simulink library "DT_Library"  (R2025b)
settings: Solver=VariableStepAuto  StartTime=0.0  StopTime=10.0  RelTol=1e-3
undefined symbols (not defined in the file or in its folder): Ala, Arg, Asn, Asp, BMedia, BRX, Choline, CMP, Glc, Glu, Gly, GMP, GSmode, His, Ile, K_ht, K_lt, Lac, Leu, Lys, mAb, Met, Phe, Pro, Ser, Thr, Trp, Tyr, V1, Val, Xv
libraries: simulink x23, $bdroot x15
(part 1 of 2)
settings Model: Creator=fenix  LastModifiedBy=Fenix

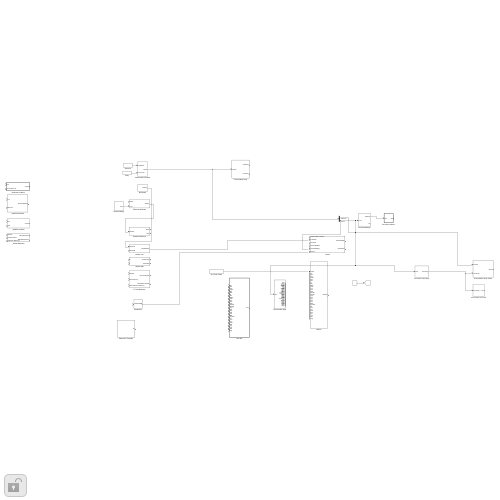
[thumbnail: Simulink's stored preview of the top-level diagram]
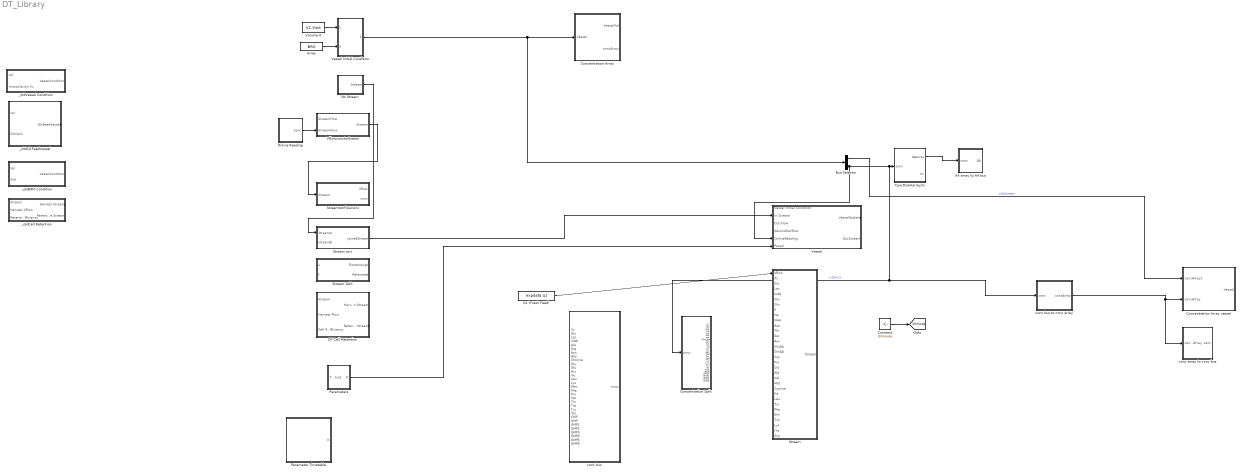
== system DT_Library ==
  AA array to AA bus : Subsystem  TreatAsAtomicUnit=on
  Array : FromWorkspace  VariableName=BRX
  Bus Selector : BusSelector  OutputSignals=Volume,conc
  Concentration Array : Subsystem
  Concentration Array vessel : Subsystem
  Concentration Split : Subsystem
  ConcttoAAarrayXv : Subsystem
  Constant : Constant  Value=GSmode
  DT Cell Retention : Subsystem
  No Stream : Subsystem
  Online Reading : Subsystem
  Parameter Timetable : Subsystem
  Parameters : Subsystem
  Q1 (Fresh Feed) : FromWorkspace  VariableName=expdata.q1  Interpolate=off  OutputAfterFinalValue=Holding final value
  Stream : Subsystem
  Stream Join : Subsystem
  Stream Split : Subsystem
  StreamtoVflowconc : Subsystem
  Vessel : Subsystem
  Vessel Initial Condition : Subsystem
  VflowconctoStream : Subsystem
  Volume 0 : Constant  Value=V1.Vinit
  _oldBRX Condition : Subsystem
  _oldCell Retention : Subsystem
  _oldGlcFeedVessel : Subsystem
  _oldVessel Condition : Subsystem  TreatAsAtomicUnit=on
  conc array to conc bus : Subsystem
  conc bus : Subsystem  TreatAsAtomicUnit=on
  conc bus to conc array : Subsystem
  tag scope: GSmode=global
  wires:
  VflowconctoStream/1(Stream) -> StreamtoVflowconc/1(Stream)
  Stream Join/1(joinedStream) -> Vessel/2(In Stream)
  No Stream/1(Stream) -> Stream Join/1(streamA)
  Array/1 -> Vessel Initial Condition/2(conc array)
  Vessel Initial Condition/1(vessel) -> Bus Selector/1, Concentration Array/1(Vessel)
  Volume 0/1 -> Vessel Initial Condition/1(VesselVol)
  Bus Selector/2 -> Vessel/5(OnlineReading), conc bus to conc array/1(conc), Concentration Split/1(conc), ConcttoAAarrayXv/1(conc)  "<conc>"
  conc bus to conc array/1(concArray) -> conc array to conc bus/1(concArray), Concentration Array vessel/2(concArray)
  Bus Selector/1 -> Concentration Array vessel/1(concArray1)  "<Volume>"
  ConcttoAAarrayXv/1(AAarray) -> AA array to AA bus/1(conc)
  Q1 (Fresh Feed)/1 -> Stream/1(Vflow)
  Parameters/1(K) -> Vessel/6(Param)
  Online Reading/1(conc) -> VflowconctoStream/2(StreamConc)
  Constant/1 -> [GSmode]

== system DT_Library/AA array to AA bus ==
  conc : Inport
  Bus Creator : BusCreator  Inputs=22  OutDataTypeStr=Bus: AA
      settings: InheritFromInputs=off
  Demux : Demux  Outputs=22
  AA : Outport
  wires:
  Demux/1 -> Bus Creator/1
  Demux/2 -> Bus Creator/2
  Demux/3 -> Bus Creator/3
  Demux/4 -> Bus Creator/4
  Demux/5 -> Bus Creator/5
  Demux/6 -> Bus Creator/6
  Demux/7 -> Bus Creator/7
  Demux/8 -> Bus Creator/8
  Demux/9 -> Bus Creator/9
  Demux/10 -> Bus Creator/10
  Demux/11 -> Bus Creator/11
  Demux/12 -> Bus Creator/12
  Demux/13 -> Bus Creator/13
  Demux/14 -> Bus Creator/14
  Demux/15 -> Bus Creator/15
  Demux/16 -> Bus Creator/16
  Demux/17 -> Bus Creator/17
  Demux/18 -> Bus Creator/18
  Demux/19 -> Bus Creator/19
  Demux/20 -> Bus Creator/20
  Demux/21 -> Bus Creator/21
  Bus Creator/1 -> AA/1
  conc/1 -> Demux/1
  Demux/22 -> Bus Creator/22

== system DT_Library/Concentration Array ==
  Vessel : Inport  OutDataTypeStr=Bus: Vessel
  Bus Selector : BusSelector  OutputSignals=Volume,conc
  conc bus to conc array : $bdroot/conc bus to conc array  SystemSampleTime=-1  VariantActivationTime=update diagram  EmptyChoice=off  PassThrough=off  PassThroughVariantControl=(default)  EmptyChoiceVariantControl=(default)  AllowFlexibleInterface=on  Latency=0  AutoFrameSizeCalculation=off
  VesselVol : Outport  OutDataTypeStr=ValueType: Volume
  concArray : Outport  Port=2
  wires:
  Bus Selector/2 -> conc bus to conc array/1  "<conc>"
  Vessel/1 -> Bus Selector/1
  Bus Selector/1 -> VesselVol/1  "<Volume>"
  conc bus to conc array/1 -> concArray/1

== system DT_Library/Concentration Array vessel ==
  concArray1 : Inport
  concArray : Inport  Port=2
  Bus Creator : BusCreator  Inputs=2  OutDataTypeStr=Bus: Vessel  NonVirtualBus=on
  conc array to conc bus : $bdroot/conc array to conc bus  SystemSampleTime=-1  VariantActivationTime=update diagram  EmptyChoice=off  PassThrough=off  PassThroughVariantControl=(default)  EmptyChoiceVariantControl=(default)  AllowFlexibleInterface=on  Latency=0  AutoFrameSizeCalculation=off
  Vessel : Outport  OutDataTypeStr=Bus: Vessel
  wires:
  concArray1/1 -> Bus Creator/1  "Volume"
  Bus Creator/1 -> Vessel/1
  concArray/1 -> conc array to conc bus/1  "concArray"
  conc array to conc bus/1 -> Bus Creator/2  "conc"

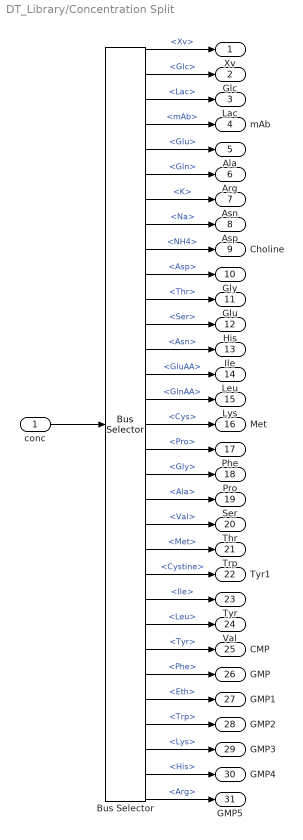
== system DT_Library/Concentration Split ==
  conc : Inport  OutDataTypeStr=Bus: conc
  Bus Selector : BusSelector  OutputSignals=Xv,Glc,Lac,mAb,Glu,Gln,K,Na,NH4,Asp,Thr,Ser,Asn,GluAA,GlnAA,Cys,Pro,Gly,Ala,Val,Met,Cystine,Ile,Leu,Tyr,Phe,Eth,Trp,Lys,His,Arg
  Xv : Outport  OutDataTypeStr=ValueType: Xvconc
  Glc : Outport  Port=2  OutDataTypeStr=ValueType: gconc
  Lac : Outport  Port=3  OutDataTypeStr=ValueType: gconc
  mAb : Outport  Port=4  OutDataTypeStr=ValueType: gconc
  Ala : Outport  Port=5  OutDataTypeStr=ValueType: mMconc
  Arg : Outport  Port=6  OutDataTypeStr=ValueType: mMconc
  Asn : Outport  Port=7  OutDataTypeStr=ValueType: mMconc
  Asp : Outport  Port=8  OutDataTypeStr=ValueType: mMconc
  Choline : Outport  Port=9  OutDataTypeStr=ValueType: mMconc
  Gly : Outport  Port=10  OutDataTypeStr=ValueType: mMconc
  Glu : Outport  Port=11  OutDataTypeStr=ValueType: mMconc
  His : Outport  Port=12  OutDataTypeStr=ValueType: mMconc
  Ile : Outport  Port=13  OutDataTypeStr=ValueType: mMconc
  Leu : Outport  Port=14  OutDataTypeStr=ValueType: mMconc
  Lys : Outport  Port=15  OutDataTypeStr=ValueType: mMconc
  Met : Outport  Port=16  OutDataTypeStr=ValueType: mMconc
  Phe : Outport  Port=17  OutDataTypeStr=ValueType: mMconc
  Pro : Outport  Port=18  OutDataTypeStr=ValueType: mMconc
  Ser : Outport  Port=19  OutDataTypeStr=ValueType: mMconc
  Thr : Outport  Port=20  OutDataTypeStr=ValueType: mMconc
  Trp : Outport  Port=21  OutDataTypeStr=ValueType: mMconc
  Tyr1 : Outport  Port=22  OutDataTypeStr=ValueType: mMconc
  Tyr : Outport  Port=23  OutDataTypeStr=ValueType: mMconc
  Val : Outport  Port=24  OutDataTypeStr=ValueType: mMconc
  CMP : Outport  Port=25  OutDataTypeStr=ValueType: mMconc
  GMP : Outport  Port=26  OutDataTypeStr=ValueType: mMconc
  GMP1 : Outport  Port=27  OutDataTypeStr=ValueType: mMconc
  GMP2 : Outport  Port=28  OutDataTypeStr=ValueType: mMconc
  GMP3 : Outport  Port=29  OutDataTypeStr=ValueType: mMconc
  GMP4 : Outport  Port=30  OutDataTypeStr=ValueType: mMconc
  GMP5 : Outport  Port=31  OutDataTypeStr=ValueType: mMconc
  wires:
  conc/1 -> Bus Selector/1
  Bus Selector/2 -> Glc/1  "<Glc>"
  Bus Selector/4 -> mAb/1  "<mAb>"
  Bus Selector/3 -> Lac/1  "<Lac>"
  Bus Selector/8 -> Asp/1  "<Na>"
  Bus Selector/16 -> Met/1  "<Cys>"
  Bus Selector/15 -> Lys/1  "<GlnAA>"
  Bus Selector/14 -> Leu/1  "<GluAA>"
  Bus Selector/13 -> Ile/1  "<Asn>"
  Bus Selector/12 -> His/1  "<Ser>"
  Bus Selector/11 -> Glu/1  "<Thr>"
  Bus Selector/10 -> Gly/1  "<Asp>"
  Bus Selector/9 -> Choline/1  "<NH4>"
  Bus Selector/5 -> Ala/1  "<Glu>"
  Bus Selector/6 -> Arg/1  "<Gln>"
  Bus Selector/7 -> Asn/1  "<K>"
  Bus Selector/21 -> Trp/1  "<Met>"
  Bus Selector/20 -> Thr/1  "<Val>"
  Bus Selector/19 -> Ser/1  "<Ala>"
  Bus Selector/18 -> Pro/1  "<Gly>"
  Bus Selector/17 -> Phe/1  "<Pro>"
  Bus Selector/1 -> Xv/1  "<Xv>"
  Bus Selector/24 -> Val/1  "<Leu>"
  Bus Selector/25 -> CMP/1  "<Tyr>"
  Bus Selector/26 -> GMP/1  "<Phe>"
  Bus Selector/23 -> Tyr/1  "<Ile>"
  Bus Selector/22 -> Tyr1/1  "<Cystine>"
  Bus Selector/27 -> GMP1/1  "<Eth>"
  Bus Selector/31 -> GMP5/1  "<Arg>"
  Bus Selector/30 -> GMP4/1  "<His>"
  Bus Selector/29 -> GMP3/1  "<Lys>"
  Bus Selector/28 -> GMP2/1  "<Trp>"

== system DT_Library/ConcttoAAarrayXv ==
  conc : Inport
  Concentration Split : $bdroot/Concentration Split  SystemSampleTime=-1  VariantActivationTime=update diagram  EmptyChoice=off  PassThrough=off  PassThroughVariantControl=(default)  EmptyChoiceVariantControl=(default)  AllowFlexibleInterface=on  Latency=0  AutoFrameSizeCalculation=off
  Mux : Mux  Inputs=22
  AAarray : Outport
  Xv : Outport  Port=2
  wires:
  conc/1 -> Concentration Split/1
  Mux/1 -> AAarray/1
  Concentration Split/1 -> Xv/1
  Concentration Split/10 -> Mux/1
  Concentration Split/11 -> Mux/2
  Concentration Split/12 -> Mux/3
  Concentration Split/13 -> Mux/4
  Concentration Split/14 -> Mux/5
  Concentration Split/15 -> Mux/6
  Concentration Split/16 -> Mux/7
  Concentration Split/17 -> Mux/8
  Concentration Split/18 -> Mux/9
  Concentration Split/19 -> Mux/10
  Concentration Split/20 -> Mux/11
  Concentration Split/21 -> Mux/12
  Concentration Split/22 -> Mux/13
  Concentration Split/23 -> Mux/14
  Concentration Split/24 -> Mux/15
  Concentration Split/25 -> Mux/16
  Concentration Split/26 -> Mux/17
  Concentration Split/27 -> Mux/18
  Concentration Split/28 -> Mux/19
  Concentration Split/29 -> Mux/20
  Concentration Split/30 -> Mux/21
  Concentration Split/31 -> Mux/22

== system DT_Library/DT Cell Retention ==
  Stream : Inport  OutDataTypeStr=Bus: Stream
  Harvest Flow : Inport  Port=2  OutDataTypeStr=ValueType: Flow
  Cell Retention Efficiency : Inport  Port=3
  CellRet : MATLAB Function  TreatAsAtomicUnit=on
  Harvest Stream : Outport  OutDataTypeStr=Bus: Stream
  Retentation Stream : Outport  Port=2  OutDataTypeStr=Bus: Stream
  wires:
  Cell Retention Efficiency/1 -> CellRet/3(RetEff)
  Harvest Flow/1 -> CellRet/2(HarvFlow)
  Stream/1 -> CellRet/1(Stream)
  CellRet/2(Ret_Stream) -> Retentation Stream/1
  CellRet/1(Harv_Stream) -> Harvest Stream/1

== system DT_Library/No Stream ==
  Stream1 : $bdroot/Stream  SystemSampleTime=-1  VariantActivationTime=update diagram  EmptyChoice=off  PassThrough=off  PassThroughVariantControl=(default)  EmptyChoiceVariantControl=(default)  AllowFlexibleInterface=on  Latency=0  AutoFrameSizeCalculation=off
  zeroXv : Constant  Value=0  OutDataTypeStr=ValueType: Xvconc
  zeroflow : Constant  Value=0  OutDataTypeStr=ValueType: Flow
  zerogconc : Constant  Value=0  OutDataTypeStr=ValueType: gconc
  zeromM : Constant  Value=0  OutDataTypeStr=ValueType: mMconc
  Stream : Outport  OutDataTypeStr=Bus: Stream
  wires:
  Stream1/1 -> Stream/1
  zeroflow/1 -> Stream1/1
  zeroXv/1 -> Stream1/2
  zerogconc/1 -> Stream1/3, Stream1/5, Stream1/4
  zeromM/1 -> Stream1/32, Stream1/31, Stream1/30, Stream1/29, Stream1/28, Stream1/27, Stream1/26, Stream1/25, Stream1/24, Stream1/23, Stream1/22, Stream1/21, Stream1/20, Stream1/19, Stream1/18, Stream1/17, Stream1/16, Stream1/15, Stream1/14, Stream1/13, Stream1/12, Stream1/11, Stream1/10, Stream1/9, Stream1/8, Stream1/7, Stream1/6

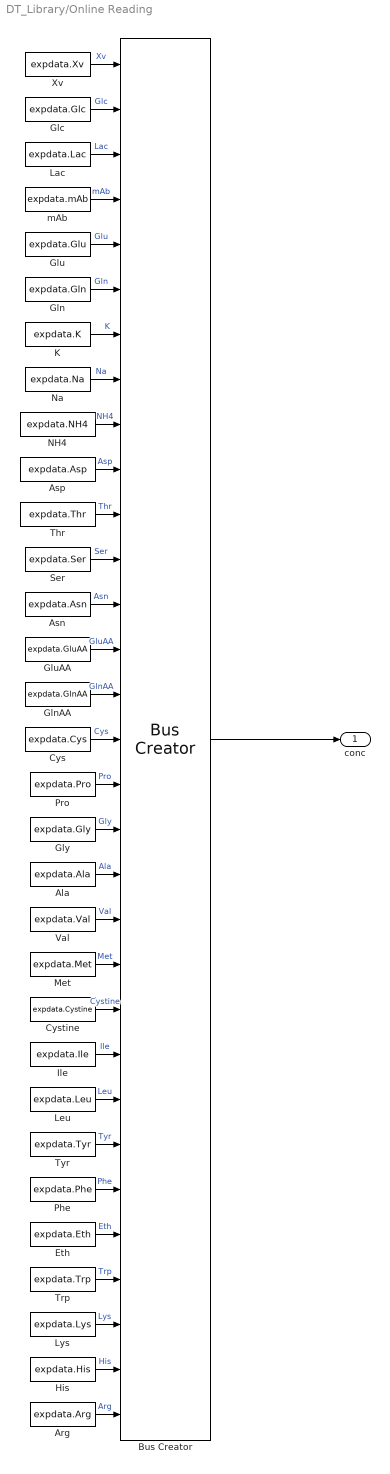
== system DT_Library/Online Reading ==
  "Ala " : FromWorkspace  VariableName=expdata.Ala
  "Arg " : FromWorkspace  VariableName=expdata.Arg
  "Asn " : FromWorkspace  VariableName=expdata.Asn
  "Asp " : FromWorkspace  VariableName=expdata.Asp
  Bus Creator : BusCreator  Inputs=31  OutDataTypeStr=Bus: conc
      settings: InheritFromInputs=off
  "Cys " : FromWorkspace  VariableName=expdata.Cys
  "Cystine " : FromWorkspace  VariableName=expdata.Cystine
  "Eth " : FromWorkspace  VariableName=expdata.Eth
  Glc : FromWorkspace  VariableName=expdata.Glc
  "Gln " : FromWorkspace  VariableName=expdata.Gln
  "GlnAA " : FromWorkspace  VariableName=expdata.GlnAA
  "Glu " : FromWorkspace  VariableName=expdata.Glu
  "GluAA " : FromWorkspace  VariableName=expdata.GluAA
  "Gly " : FromWorkspace  VariableName=expdata.Gly
  "His " : FromWorkspace  VariableName=expdata.His
  "Ile " : FromWorkspace  VariableName=expdata.Ile
  "K " : FromWorkspace  VariableName=expdata.K
  Lac : FromWorkspace  VariableName=expdata.Lac
  "Leu " : FromWorkspace  VariableName=expdata.Leu
  "Lys " : FromWorkspace  VariableName=expdata.Lys
  "Met " : FromWorkspace  VariableName=expdata.Met
  "NH4 " : FromWorkspace  VariableName=expdata.NH4
  "Na " : FromWorkspace  VariableName=expdata.Na
  Phe : FromWorkspace  VariableName=expdata.Phe
  "Pro " : FromWorkspace  VariableName=expdata.Pro
  "Ser " : FromWorkspace  VariableName=expdata.Ser
  "Thr " : FromWorkspace  VariableName=expdata.Thr
  "Trp " : FromWorkspace  VariableName=expdata.Trp
  Tyr : FromWorkspace  VariableName=expdata.Tyr
  "Val " : FromWorkspace  VariableName=expdata.Val
  Xv : FromWorkspace  VariableName=expdata.Xv
  mAb : FromWorkspace  VariableName=expdata.mAb
  conc : Outport  OutDataTypeStr=Bus: conc
  wires:
  "Glu "/1 -> Bus Creator/5  "Glu"
  "Gln "/1 -> Bus Creator/6  "Gln"
  "K "/1 -> Bus Creator/7  "K"
  "Na "/1 -> Bus Creator/8  "Na"
  Xv/1 -> Bus Creator/1  "Xv"
  Glc/1 -> Bus Creator/2  "Glc"
  Lac/1 -> Bus Creator/3  "Lac"
  mAb/1 -> Bus Creator/4  "mAb"
  Bus Creator/1 -> conc/1
  "NH4 "/1 -> Bus Creator/9  "NH4"
  "Asp "/1 -> Bus Creator/10  "Asp"
  "Thr "/1 -> Bus Creator/11  "Thr"
  "Asn "/1 -> Bus Creator/13  "Asn"
  "Ser "/1 -> Bus Creator/12  "Ser"
  "Eth "/1 -> Bus Creator/27  "Eth"
  Phe/1 -> Bus Creator/26  "Phe"
  Tyr/1 -> Bus Creator/25  "Tyr"
  "Leu "/1 -> Bus Creator/24  "Leu"
  "Ile "/1 -> Bus Creator/23  "Ile"
  "Cystine "/1 -> Bus Creator/22  "Cystine"
  "Met "/1 -> Bus Creator/21  "Met"
  "Val "/1 -> Bus Creator/20  "Val"
  "Ala "/1 -> Bus Creator/19  "Ala"
  "Gly "/1 -> Bus Creator/18  "Gly"
  "Pro "/1 -> Bus Creator/17  "Pro"
  "Cys "/1 -> Bus Creator/16  "Cys"
  "GlnAA "/1 -> Bus Creator/15  "GlnAA"
  "GluAA "/1 -> Bus Creator/14  "GluAA"
  "Arg "/1 -> Bus Creator/31  "Arg"
  "His "/1 -> Bus Creator/30  "His"
  "Lys "/1 -> Bus Creator/29  "Lys"
  "Trp "/1 -> Bus Creator/28  "Trp"

== system DT_Library/Parameter Timetable ==
  From Workspace : FromWorkspace  VariableName=KTT.Ylacglc  Interpolate=off  OutputAfterFinalValue=Holding final value
  From Workspace1 : FromWorkspace  VariableName=KTT.Ymabxv  OutputAfterFinalValue=Holding final value
  From Workspace2 : FromWorkspace  VariableName=KTT.Yxvglc  OutputAfterFinalValue=Holding final value
  From Workspace3 : FromWorkspace  VariableName=KTT.kdlac  OutputAfterFinalValue=Holding final value
  From Workspace4 : FromWorkspace  VariableName=KTT.kglc  OutputAfterFinalValue=Holding final value
  From Workspace5 : FromWorkspace  VariableName=KTT.kilac  OutputAfterFinalValue=Holding final value
  From Workspace6 : FromWorkspace  VariableName=KTT.mglc  OutputAfterFinalValue=Holding final value
  From Workspace7 : FromWorkspace  VariableName=KTT.udmax
  From Workspace8 : FromWorkspace  VariableName=KTT.umax  OutputAfterFinalValue=Holding final value
  From Workspace9 : FromWorkspace  VariableName=KTT.Yxvlac  OutputAfterFinalValue=Holding final value
  parameter bus : $bdroot/Parameters/parameter bus  SystemSampleTime=-1  VariantActivationTime=update diagram  EmptyChoice=off  PassThrough=off  PassThroughVariantControl=(default)  EmptyChoiceVariantControl=(default)  AllowFlexibleInterface=on  Latency=0  AutoFrameSizeCalculation=off
  K : Outport
  wires:
  From Workspace2/1 -> parameter bus/3
  From Workspace9/1 -> parameter bus/10
  From Workspace/1 -> parameter bus/1
  From Workspace3/1 -> parameter bus/4
  From Workspace1/1 -> parameter bus/2
  From Workspace6/1 -> parameter bus/7
  From Workspace4/1 -> parameter bus/5
  From Workspace8/1 -> parameter bus/9
  From Workspace5/1 -> parameter bus/6
  From Workspace7/1 -> parameter bus/8
  parameter bus/1 -> K/1

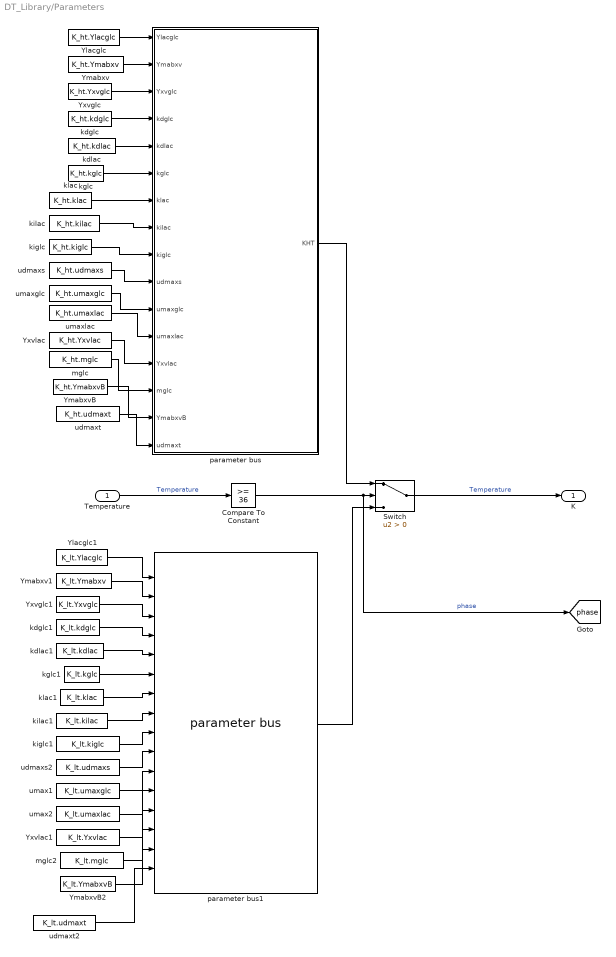
== system DT_Library/Parameters ==
  Temperature : Inport
  Compare To Constant : simulink/Logic and Bit Operations/Compare To Constant  relop=>=  const=36  OutDataTypeStr=boolean
  Switch : Switch  Criteria=u2 > Threshold  ZeroCross=off  SaturateOnIntegerOverflow=off  InputSameDT=off
  Ylacglc : Constant  Value=K_ht.Ylacglc
  Ylacglc1 : Constant  Value=K_lt.Ylacglc
  Ymabxv : Constant  Value=K_ht.Ymabxv
  Ymabxv1 : Constant  Value=K_lt.Ymabxv
  YmabxvB : Constant  Value=K_ht.YmabxvB
  YmabxvB2 : Constant  Value=K_lt.YmabxvB
  Yxvglc : Constant  Value=K_ht.Yxvglc
  Yxvglc1 : Constant  Value=K_lt.Yxvglc
  Yxvlac : Constant  Value=K_ht.Yxvlac
  Yxvlac1 : Constant  Value=K_lt.Yxvlac
  kdglc : Constant  Value=K_ht.kdglc
  kdglc1 : Constant  Value=K_lt.kdglc
  kdlac : Constant  Value=K_ht.kdlac
  kdlac1 : Constant  Value=K_lt.kdlac
  kglc : Constant  Value=K_ht.kglc
  kglc1 : Constant  Value=K_lt.kglc
  kiglc : Constant  Value=K_ht.kiglc
  kiglc1 : Constant  Value=K_lt.kiglc
  kilac : Constant  Value=K_ht.kilac
  kilac1 : Constant  Value=K_lt.kilac
  klac : Constant  Value=K_ht.klac
  klac1 : Constant  Value=K_lt.klac
  mglc : Constant  Value=K_ht.mglc
  mglc2 : Constant  Value=K_lt.mglc
  parameter bus : Subsystem  TreatAsAtomicUnit=on
  parameter bus1 : $bdroot/Parameters/parameter bus  SystemSampleTime=-1  VariantActivationTime=update diagram  EmptyChoice=off  PassThrough=off  PassThroughVariantControl=(default)  EmptyChoiceVariantControl=(default)  AllowFlexibleInterface=on  Latency=0  AutoFrameSizeCalculation=off
  udmaxs : Constant  Value=K_ht.udmaxs
  udmaxs2 : Constant  Value=K_lt.udmaxs
  udmaxt : Constant  Value=K_ht.udmaxt
  udmaxt2 : Constant  Value=K_lt.udmaxt
  umax1 : Constant  Value=K_lt.umaxglc
  umax2 : Constant  Value=K_lt.umaxlac
  umaxglc : Constant  Value=K_ht.umaxglc
  umaxlac : Constant  Value=K_ht.umaxlac
  K : Outport
  tag scope: phase=global
  wires:
  parameter bus/1(KHT) -> Switch/1
  kdlac/1 -> parameter bus/5(kdlac)
  Ylacglc/1 -> parameter bus/1(Ylacglc)
  kglc/1 -> parameter bus/6(kglc)
  Ymabxv/1 -> parameter bus/2(Ymabxv)
  klac/1 -> parameter bus/7(klac)
  Yxvglc/1 -> parameter bus/3(Yxvglc)
  kilac/1 -> parameter bus/8(kilac)
  kdglc/1 -> parameter bus/4(kdglc)
  kiglc/1 -> parameter bus/9(kiglc)
  Temperature/1 -> Compare To Constant/1  "Temperature"
  Compare To Constant/1 -> [phase], Switch/2  "phase"
  parameter bus1/1 -> Switch/3
  Switch/1 -> K/1  "Temperature"
  udmaxs/1 -> parameter bus/10(udmaxs)
  umaxglc/1 -> parameter bus/11(umaxglc)
  umaxlac/1 -> parameter bus/12(umaxlac)
  Ylacglc1/1 -> parameter bus1/1
  Ymabxv1/1 -> parameter bus1/2
  Yxvglc1/1 -> parameter bus1/3
  kdglc1/1 -> parameter bus1/4
  kdlac1/1 -> parameter bus1/5
  kglc1/1 -> parameter bus1/6
  kilac1/1 -> parameter bus1/8
  klac1/1 -> parameter bus1/7
  kiglc1/1 -> parameter bus1/9
  udmaxs2/1 -> parameter bus1/10
  umax1/1 -> parameter bus1/11
  Yxvlac/1 -> parameter bus/13(Yxvlac)
  mglc/1 -> parameter bus/14(mglc)
  YmabxvB/1 -> parameter bus/15(YmabxvB)
  Yxvlac1/1 -> parameter bus1/13
  umax2/1 -> parameter bus1/12
  YmabxvB2/1 -> parameter bus1/15
  mglc2/1 -> parameter bus1/14
  udmaxt2/1 -> parameter bus1/16
  udmaxt/1 -> parameter bus/16(udmaxt)

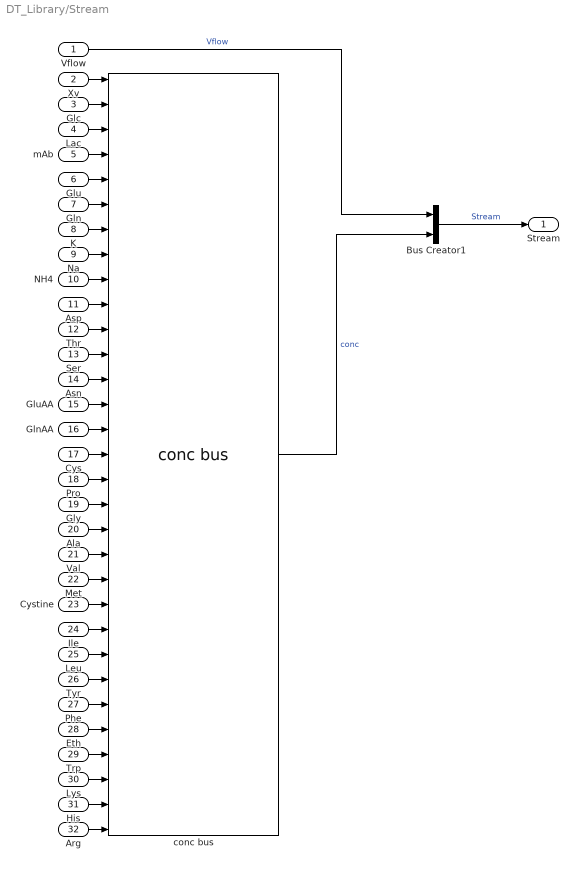
== system DT_Library/Stream ==
  Vflow : Inport  OutDataTypeStr=ValueType: Flow
  "Xv " : Inport  Port=2  OutDataTypeStr=ValueType: Xvconc
  "Glc " : Inport  Port=3  OutDataTypeStr=ValueType: gconc
  "Lac " : Inport  Port=4  OutDataTypeStr=ValueType: gconc
  mAb : Inport  Port=5  OutDataTypeStr=ValueType: gconc
  "Glu " : Inport  Port=6  OutDataTypeStr=ValueType: mMconc
  "Gln " : Inport  Port=7  OutDataTypeStr=ValueType: mMconc
  "K " : Inport  Port=8  OutDataTypeStr=ValueType: mMconc
  "Na " : Inport  Port=9  OutDataTypeStr=ValueType: mMconc
  "NH4 " : Inport  Port=10  OutDataTypeStr=ValueType: mMconc
  "Asp " : Inport  Port=11  OutDataTypeStr=ValueType: mMconc
  "Thr " : Inport  Port=12  OutDataTypeStr=ValueType: mMconc
  "Ser " : Inport  Port=13  OutDataTypeStr=ValueType: mMconc
  "Asn " : Inport  Port=14  OutDataTypeStr=ValueType: mMconc
  "GluAA " : Inport  Port=15  OutDataTypeStr=ValueType: mMconc
  "GlnAA " : Inport  Port=16  OutDataTypeStr=ValueType: mMconc
  "Cys " : Inport  Port=17  OutDataTypeStr=ValueType: mMconc
  "Pro " : Inport  Port=18  OutDataTypeStr=ValueType: mMconc
  "Gly " : Inport  Port=19  OutDataTypeStr=ValueType: mMconc
  "Ala " : Inport  Port=20  OutDataTypeStr=ValueType: mMconc
  "Val " : Inport  Port=21  OutDataTypeStr=ValueType: mMconc
  "Met " : Inport  Port=22  OutDataTypeStr=ValueType: mMconc
  "Cystine " : Inport  Port=23  OutDataTypeStr=ValueType: mMconc
  "Ile " : Inport  Port=24  OutDataTypeStr=ValueType: mMconc
  "Leu " : Inport  Port=25  OutDataTypeStr=ValueType: mMconc
  "Tyr " : Inport  Port=26  OutDataTypeStr=ValueType: mMconc
  "Phe " : Inport  Port=27  OutDataTypeStr=ValueType: mMconc
  "Eth " : Inport  Port=28  OutDataTypeStr=ValueType: mMconc
  "Trp " : Inport  Port=29  OutDataTypeStr=ValueType: mMconc
  "Lys " : Inport  Port=30  OutDataTypeStr=ValueType: mMconc
  "His " : Inport  Port=31  OutDataTypeStr=ValueType: mMconc
  "Arg " : Inport  Port=32  OutDataTypeStr=ValueType: mMconc
  Bus Creator1 : BusCreator  Inputs=2  OutDataTypeStr=Bus: Stream
      settings: InheritFromInputs=off
  conc bus : $bdroot/conc bus  SystemSampleTime=-1  VariantActivationTime=update diagram  EmptyChoice=off  PassThrough=off  PassThroughVariantControl=(default)  EmptyChoiceVariantControl=(default)  AllowFlexibleInterface=on  Latency=0  AutoFrameSizeCalculation=off
  Stream : Outport  OutDataTypeStr=Bus: Stream
  wires:
  Vflow/1 -> Bus Creator1/1  "Vflow"
  Bus Creator1/1 -> Stream/1  "Stream"
  conc bus/1 -> Bus Creator1/2  "conc"
  "Xv "/1 -> conc bus/1
  "Lac "/1 -> conc bus/3
  "Glc "/1 -> conc bus/2
  mAb/1 -> conc bus/4
  "Glu "/1 -> conc bus/5
  "Gln "/1 -> conc bus/6
  "Ala "/1 -> conc bus/19
  "Arg "/1 -> conc bus/31
  "His "/1 -> conc bus/30
  "Lys "/1 -> conc bus/29
  "Trp "/1 -> conc bus/28
  "Eth "/1 -> conc bus/27
  "Phe "/1 -> conc bus/26
  "Tyr "/1 -> conc bus/25
  "Leu "/1 -> conc bus/24
  "Ile "/1 -> conc bus/23
  "Cystine "/1 -> conc bus/22
  "Met "/1 -> conc bus/21
  "Val "/1 -> conc bus/20
  "Gly "/1 -> conc bus/18
  "Pro "/1 -> conc bus/17
  "Cys "/1 -> conc bus/16
  "GlnAA "/1 -> conc bus/15
  "GluAA "/1 -> conc bus/14
  "Asn "/1 -> conc bus/13
  "Ser "/1 -> conc bus/12
  "Thr "/1 -> conc bus/11
  "Asp "/1 -> conc bus/10
  "NH4 "/1 -> conc bus/9
  "Na "/1 -> conc bus/8
  "K "/1 -> conc bus/7

== system DT_Library/Stream Join ==
  streamA : Inport  OutDataTypeStr=Bus: Stream
  streamB : Inport  Port=2  OutDataTypeStr=Bus: Stream
  MATLAB Function : MATLAB Function  TreatAsAtomicUnit=on
  joinedStream : Outport  OutDataTypeStr=Bus: Stream
  wires:
  streamB/1 -> MATLAB Function/2(B)
  streamA/1 -> MATLAB Function/1(A)
  MATLAB Function/1(joinedstream) -> joinedStream/1

== system DT_Library/Stream Split ==
  u : Inport  OutDataTypeStr=Bus: Stream
  f : Inport  Port=2  OutDataTypeStr=Bus: Stream
  MATLAB Function : MATLAB Function  TreatAsAtomicUnit=on
  Flowthrough : Outport  OutDataTypeStr=Bus: Stream
  Retentate : Outport  Port=2  OutDataTypeStr=Bus: Stream
  wires:
  MATLAB Function/1(Flowthrough) -> Flowthrough/1
  MATLAB Function/2(Retentate) -> Retentate/1
  u/1 -> MATLAB Function/1(u)
  f/1 -> MATLAB Function/2(f)

== system DT_Library/StreamtoVflowconc ==
  Stream : Inport  OutDataTypeStr=Bus: Stream
  Bus Selector : BusSelector  OutputSignals=Vflow,conc
  Vflow : Outport  OutDataTypeStr=ValueType: Flow
  conc : Outport  Port=2  OutDataTypeStr=Bus: conc
  wires:
  Stream/1 -> Bus Selector/1
  Bus Selector/1 -> Vflow/1  "<Vflow>"
  Bus Selector/2 -> conc/1  "<conc>"

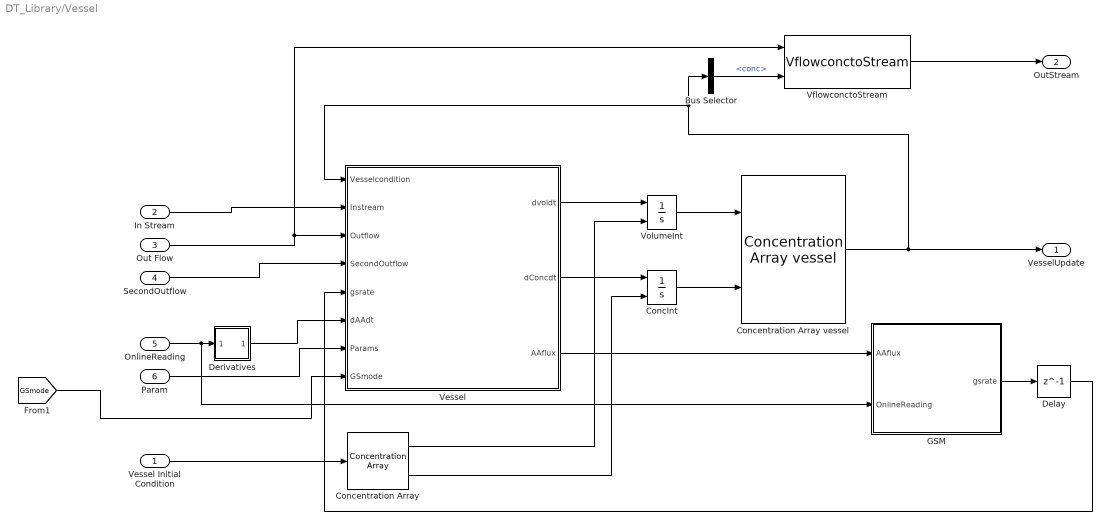
== system DT_Library/Vessel ==
  Vessel Initial Condition : Inport  OutDataTypeStr=Bus: Vessel
  In Stream : Inport  Port=2  OutDataTypeStr=Bus: Stream
  Out Flow : Inport  Port=3  OutDataTypeStr=ValueType: Flow
  SecondOutflow : Inport  Port=4  OutDataTypeStr=ValueType: Flow
  OnlineReading : Inport  Port=5  OutDataTypeStr=Bus: conc
  Param : Inport  Port=6  OutDataTypeStr=Bus: K
  Bus Selector : BusSelector  OutputSignals=conc
  ConcInt : Integrator  InitialConditionSource=external  LimitOutput=on  LowerSaturationLimit=0
  Concentration Array : $bdroot/Concentration Array  SystemSampleTime=-1  VariantActivationTime=update diagram  EmptyChoice=off  PassThrough=off  PassThroughVariantControl=(default)  EmptyChoiceVariantControl=(default)  AllowFlexibleInterface=on  Latency=0  AutoFrameSizeCalculation=off
  Concentration Array vessel : $bdroot/Concentration Array vessel  SystemSampleTime=-1  VariantActivationTime=update diagram  EmptyChoice=off  PassThrough=off  PassThroughVariantControl=(default)  EmptyChoiceVariantControl=(default)  AllowFlexibleInterface=on  Latency=0  AutoFrameSizeCalculation=off
  Delay : Delay  DelayLength=1
  Derivatives : Subsystem
  GSM : Subsystem
  Vessel : MATLAB Function  TreatAsAtomicUnit=on
  VflowconctoStream : $bdroot/VflowconctoStream  SystemSampleTime=-1  VariantActivationTime=update diagram  EmptyChoice=off  PassThrough=off  PassThroughVariantControl=(default)  EmptyChoiceVariantControl=(default)  AllowFlexibleInterface=on  Latency=0  AutoFrameSizeCalculation=off
  VolumeInt : Integrator  InitialConditionSource=external  LimitOutput=on  LowerSaturationLimit=0
  VesselUpdate : Outport  OutDataTypeStr=Bus: Vessel
  OutStream : Outport  Port=2  OutDataTypeStr=Bus: Stream
  wires:
  Vessel Initial Condition/1 -> Concentration Array/1
  Out Flow/1 -> VflowconctoStream/1, Vessel/3(Outflow)
  In Stream/1 -> Vessel/2(Instream)
  Vessel/1(dvoldt) -> VolumeInt/1
  Vessel/2(dConcdt) -> ConcInt/1
  VolumeInt/1 -> Concentration Array vessel/1
  ConcInt/1 -> Concentration Array vessel/2
  Concentration Array/1 -> VolumeInt/2
  Concentration Array/2 -> ConcInt/2
  VflowconctoStream/1 -> OutStream/1
  Bus Selector/1 -> VflowconctoStream/2  "<conc>"
  SecondOutflow/1 -> Vessel/4(SecondOutflow)
  Concentration Array vessel/1 -> VesselUpdate/1, Bus Selector/1, Vessel/1(Vesselcondition)
  OnlineReading/1 -> GSM/2(OnlineReading), Derivatives/1(OnlineReading)
  GSM/1(gsrate) -> Delay/1
  Delay/1 -> Vessel/5(gsrate)
  Derivatives/1(dAAdt) -> Vessel/6(dAAdt)
  Vessel/3(AAflux) -> GSM/1(AAflux)
  Param/1 -> Vessel/7(Params)
  [GSmode] -> Vessel/8(GSmode)

== system DT_Library/Vessel Initial Condition ==
  VesselVol : Inport  OutDataTypeStr=ValueType: Volume
  conc array : Inport  Port=2
  Bus Creator : BusCreator  Inputs=2  OutDataTypeStr=Bus: Vessel
      settings: InheritFromInputs=off
  conc array to conc bus : $bdroot/conc array to conc bus  SystemSampleTime=-1  VariantActivationTime=update diagram  EmptyChoice=off  PassThrough=off  PassThroughVariantControl=(default)  EmptyChoiceVariantControl=(default)  AllowFlexibleInterface=on  Latency=0  AutoFrameSizeCalculation=off
  vessel : Outport
  wires:
  Bus Creator/1 -> vessel/1
  VesselVol/1 -> Bus Creator/1  "Volume"
  conc array/1 -> conc array to conc bus/1
  conc array to conc bus/1 -> Bus Creator/2  "conc"

== system DT_Library/VflowconctoStream ==
  StreamFlow : Inport  OutDataTypeStr=ValueType: Flow
  StreamConc : Inport  Port=2  OutDataTypeStr=Bus: conc
  Bus Creator : BusCreator  Inputs=2  OutDataTypeStr=Bus: Stream
  Stream : Outport  OutDataTypeStr=Bus: Stream
  wires:
  StreamFlow/1 -> Bus Creator/1  "Vflow"
  StreamConc/1 -> Bus Creator/2  "conc"
  Bus Creator/1 -> Stream/1

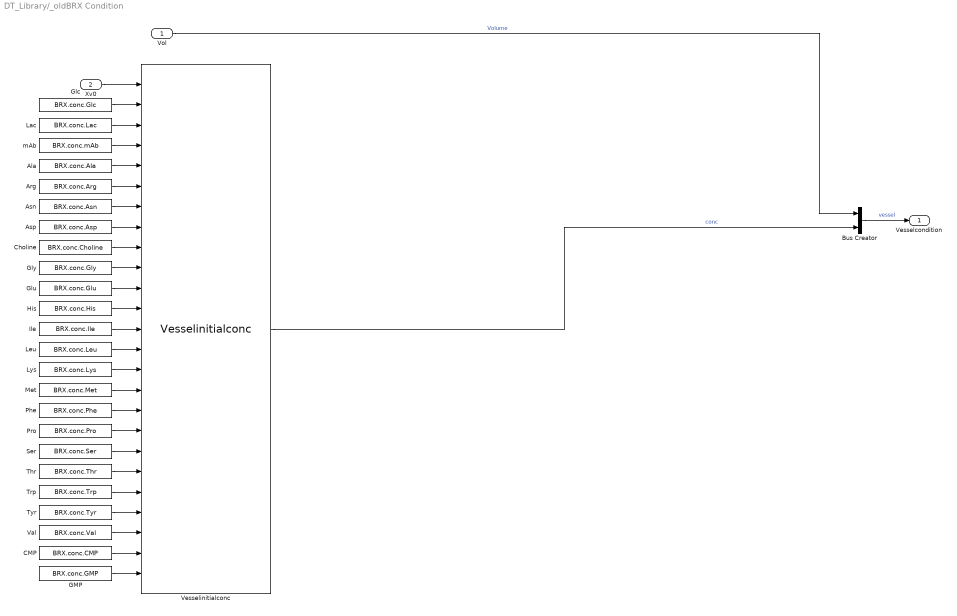
== system DT_Library/_oldBRX Condition ==
  Vol : Inport
  Xv0 : Inport  Port=2
  Ala : Constant  Value=BRX.conc.Ala  OutDataTypeStr=ValueType: mMconc
  Arg : Constant  Value=BRX.conc.Arg  OutDataTypeStr=ValueType: mMconc
  Asn : Constant  Value=BRX.conc.Asn  OutDataTypeStr=ValueType: mMconc
  Asp : Constant  Value=BRX.conc.Asp  OutDataTypeStr=ValueType: mMconc
  Bus Creator : BusCreator  Inputs=2
  CMP : Constant  Value=BRX.conc.CMP  OutDataTypeStr=ValueType: mMconc
  Choline : Constant  Value=BRX.conc.Choline  OutDataTypeStr=ValueType: mMconc
  GMP : Constant  Value=BRX.conc.GMP  OutDataTypeStr=ValueType: mMconc
  Glc : Constant  Value=BRX.conc.Glc  OutDataTypeStr=ValueType: gconc
  Glu : Constant  Value=BRX.conc.Glu  OutDataTypeStr=ValueType: mMconc
  Gly : Constant  Value=BRX.conc.Gly  OutDataTypeStr=ValueType: mMconc
  His : Constant  Value=BRX.conc.His  OutDataTypeStr=ValueType: mMconc
  Ile : Constant  Value=BRX.conc.Ile  OutDataTypeStr=ValueType: mMconc
  Lac : Constant  Value=BRX.conc.Lac  OutDataTypeStr=ValueType: gconc
  Leu : Constant  Value=BRX.conc.Leu  OutDataTypeStr=ValueType: mMconc
  Lys : Constant  Value=BRX.conc.Lys  OutDataTypeStr=ValueType: mMconc
  Met : Constant  Value=BRX.conc.Met  OutDataTypeStr=ValueType: mMconc
  Phe : Constant  Value=BRX.conc.Phe  OutDataTypeStr=ValueType: mMconc
  Pro : Constant  Value=BRX.conc.Pro  OutDataTypeStr=ValueType: mMconc
  Ser : Constant  Value=BRX.conc.Ser  OutDataTypeStr=ValueType: mMconc
  Thr : Constant  Value=BRX.conc.Thr  OutDataTypeStr=ValueType: mMconc
  Trp : Constant  Value=BRX.conc.Trp  OutDataTypeStr=ValueType: mMconc
  Tyr : Constant  Value=BRX.conc.Tyr  OutDataTypeStr=ValueType: mMconc
  Val : Constant  Value=BRX.conc.Val  OutDataTypeStr=ValueType: mMconc
  Vesselinitialconc : $bdroot/Vessel Condition/Initial Concentration/Vesselinitialconc  SystemSampleTime=-1  VariantActivationTime=update diagram  EmptyChoice=off  PassThrough=off  PassThroughVariantControl=(default)  EmptyChoiceVariantControl=(default)  AllowFlexibleInterface=on  Latency=0  AutoFrameSizeCalculation=off
      link override Bus Creator: Inputs=25
  mAb : Constant  Value=BRX.conc.mAb  OutDataTypeStr=ValueType: gconc
  Vesselcondition : Outport  OutDataTypeStr=Bus: Vessel
  wires:
  Xv0/1 -> Vesselinitialconc/1
  Glc/1 -> Vesselinitialconc/2
  Lac/1 -> Vesselinitialconc/3
  mAb/1 -> Vesselinitialconc/4
  Ala/1 -> Vesselinitialconc/5
  Arg/1 -> Vesselinitialconc/6
  Asn/1 -> Vesselinitialconc/7
  Asp/1 -> Vesselinitialconc/8
  Choline/1 -> Vesselinitialconc/9
  Gly/1 -> Vesselinitialconc/10
  Glu/1 -> Vesselinitialconc/11
  His/1 -> Vesselinitialconc/12
  Ile/1 -> Vesselinitialconc/13
  Leu/1 -> Vesselinitialconc/14
  Lys/1 -> Vesselinitialconc/15
  Met/1 -> Vesselinitialconc/16
  Phe/1 -> Vesselinitialconc/17
  Pro/1 -> Vesselinitialconc/18
  Ser/1 -> Vesselinitialconc/19
  Thr/1 -> Vesselinitialconc/20
  Trp/1 -> Vesselinitialconc/21
  Tyr/1 -> Vesselinitialconc/22
  Val/1 -> Vesselinitialconc/23
  CMP/1 -> Vesselinitialconc/24
  GMP/1 -> Vesselinitialconc/25
  Vol/1 -> Bus Creator/1  "Volume"
  Vesselinitialconc/1 -> Bus Creator/2  "conc"
  Bus Creator/1 -> Vesselcondition/1  "vessel"

== system DT_Library/_oldCell Retention ==
  Stream : Inport  OutDataTypeStr=Bus: Stream
  Harvest VFlow : Inport  Port=2  OutDataTypeStr=ValueType: Flow
  Retention Efficiency : Inport  Port=3
  Bus Assignment : BusAssignment  AssignedSignals=Xv
  Bus Assignment1 : BusAssignment  AssignedSignals=Xv
  Bus Selector : BusSelector  OutputSignals=Xv
  Bus Selector1 : BusSelector  OutputSignals=Vflow,conc
  Divide : Product  Inputs=/*
  HarvStream : BusCreator  Inputs=2  OutDataTypeStr=Bus: Stream
      settings: InheritFromInputs=off
  HarvestXv : Product  Inputs=/*
  Product : Product
  Product1 : Product
  RetStream : BusCreator  Inputs=2  OutDataTypeStr=Bus: Stream
  RetVflow : Sum  Inputs=+-
  Subtract : Sum  Inputs=+-
  Harvest Stream : Outport  OutDataTypeStr=Bus: Stream
  Retentate Stream : Outport  Port=2  OutDataTypeStr=Bus: Stream
  wires:
  Bus Assignment/1 -> HarvStream/2  "conc"
  Bus Assignment1/1 -> RetStream/2  "conc"
  Stream/1 -> Bus Selector1/1
  Retention Efficiency/1 -> Product1/2
  Harvest VFlow/1 -> HarvStream/1, HarvestXv/1, RetVflow/2  "Vflow"
  Bus Selector1/2 -> Bus Assignment/1, Bus Assignment1/1, Bus Selector/1  "<conc>"
  HarvStream/1 -> Harvest Stream/1  "Harvest"
  RetStream/1 -> Retentate Stream/1  "Retentate"
  Bus Selector1/1 -> Product/1, RetVflow/1  "<Vflow>"
  HarvestXv/1 -> Bus Assignment/2
  Divide/1 -> Bus Assignment1/2
  Product1/1 -> Subtract/2, Divide/2
  Product/1 -> Subtract/1, Product1/1
  Subtract/1 -> HarvestXv/2
  RetVflow/1 -> RetStream/1, Divide/1  "Vflow"
  Bus Selector/1 -> Product/2  "<Xv>"

== system DT_Library/_oldGlcFeedVessel ==
  vol : Inport
  GlcConc : Inport  Port=2
  Bus Assignment : BusAssignment  AssignedSignals=conc
  Bus Assignment1 : BusAssignment  AssignedSignals=conc.Glc
  Bus Selector : BusSelector  OutputSignals=conc
  Constant2 : Constant  Value=0
  No Stream1 : $bdroot/No Stream  SystemSampleTime=-1  VariantActivationTime=update diagram  EmptyChoice=off  PassThrough=off  PassThroughVariantControl=(default)  EmptyChoiceVariantControl=(default)  AllowFlexibleInterface=on  Latency=0  AutoFrameSizeCalculation=off
  Vessel Condition1 : $bdroot/Vessel Condition  SystemSampleTime=-1  VariantActivationTime=update diagram  EmptyChoice=off  PassThrough=off  PassThroughVariantControl=(default)  EmptyChoiceVariantControl=(default)  AllowFlexibleInterface=on  Latency=0  AutoFrameSizeCalculation=off
  GlcFeedVessel : Outport
  wires:
  GlcConc/1 -> Bus Assignment1/2
  Bus Assignment/1 -> Bus Assignment1/1
  Bus Selector/1 -> Bus Assignment/2  "<conc>"
  vol/1 -> Vessel Condition1/1
  Constant2/1 -> Vessel Condition1/2
  Vessel Condition1/1 -> Bus Assignment/1
  No Stream1/1 -> Bus Selector/1
  Bus Assignment1/1 -> GlcFeedVessel/1

== system DT_Library/_oldVessel Condition ==
  vol : Inport  OutDataTypeStr=ValueType: Volume
  Innoculation Xv : Inport  Port=2  OutDataTypeStr=ValueType: Xvconc
  Bus Creator : BusCreator  Inputs=2
  Initial Concentration : Subsystem
  Vesselcondition : Outport  OutDataTypeStr=Bus: Vessel
  wires:
  Innoculation Xv/1 -> Initial Concentration/1(Xv)
  Initial Concentration/1(conc) -> Bus Creator/2  "conc"
  vol/1 -> Bus Creator/1  "Volume"
  Bus Creator/1 -> Vesselcondition/1  "vessel"

== system DT_Library/conc array to conc bus ==
  concArray : Inport
  Bus Creator : BusCreator  Inputs=31  OutDataTypeStr=Bus: conc  NonVirtualBus=on
      settings: InheritFromInputs=off
  Demux : Demux  Outputs=31
  conc : Outport
  wires:
  concArray/1 -> Demux/1
  Demux/1 -> Bus Creator/1  "Xv"
  Demux/2 -> Bus Creator/2  "Glc"
  Demux/3 -> Bus Creator/3  "Lac"
  Demux/4 -> Bus Creator/4  "mAb"
  Demux/5 -> Bus Creator/5  "Glu"
  Demux/6 -> Bus Creator/6  "Gln"
  Demux/7 -> Bus Creator/7  "K"
  Demux/8 -> Bus Creator/8  "Na"
  Demux/9 -> Bus Creator/9  "NH4"
  Demux/10 -> Bus Creator/10  "Asp"
  Demux/11 -> Bus Creator/11  "Thr"
  Demux/12 -> Bus Creator/12  "Ser"
  Demux/13 -> Bus Creator/13  "Asn"
  Demux/14 -> Bus Creator/14  "GluAA"
  Demux/15 -> Bus Creator/15  "GlnAA"
  Demux/16 -> Bus Creator/16  "Cys"
  Demux/17 -> Bus Creator/17  "Pro"
  Demux/18 -> Bus Creator/18  "Gly"
  Demux/19 -> Bus Creator/19  "Ala"
  Demux/20 -> Bus Creator/20  "Val"
  Demux/21 -> Bus Creator/21  "Met"
  Demux/22 -> Bus Creator/22  "Cystine"
  Demux/23 -> Bus Creator/23  "Ile"
  Demux/24 -> Bus Creator/24  "Leu"
  Demux/25 -> Bus Creator/25  "Tyr"
  Demux/26 -> Bus Creator/26  "Phe"
  Demux/27 -> Bus Creator/27  "Eth"
  Bus Creator/1 -> conc/1
  Demux/28 -> Bus Creator/28  "Trp"
  Demux/29 -> Bus Creator/29  "Lys"
  Demux/30 -> Bus Creator/30  "His"
  Demux/31 -> Bus Creator/31  "Arg"

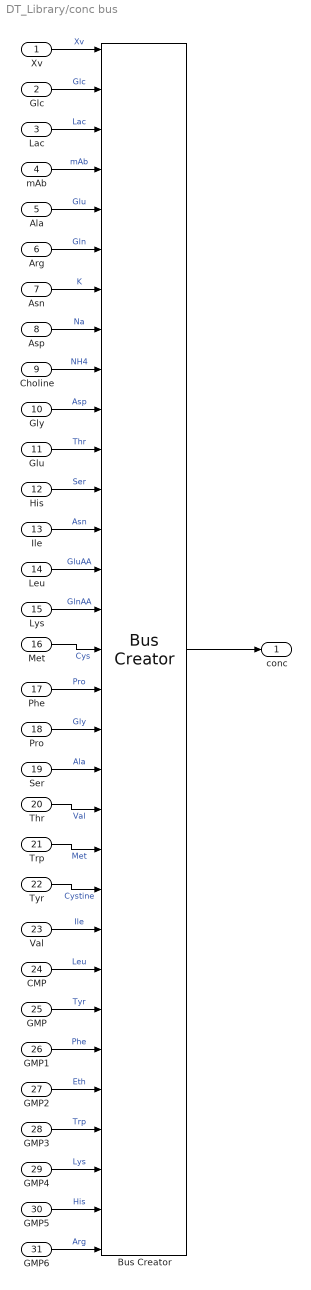
== system DT_Library/conc bus ==
  Xv : Inport  OutDataTypeStr=ValueType: Xvconc
  Glc : Inport  Port=2  OutDataTypeStr=ValueType: gconc
  Lac : Inport  Port=3  OutDataTypeStr=ValueType: gconc
  mAb : Inport  Port=4  OutDataTypeStr=ValueType: gconc
  Ala : Inport  Port=5  OutDataTypeStr=ValueType: mMconc
  Arg : Inport  Port=6  OutDataTypeStr=ValueType: mMconc
  Asn : Inport  Port=7  OutDataTypeStr=ValueType: mMconc
  Asp : Inport  Port=8  OutDataTypeStr=ValueType: mMconc
  Choline : Inport  Port=9  OutDataTypeStr=ValueType: mMconc
  Gly : Inport  Port=10  OutDataTypeStr=ValueType: mMconc
  Glu : Inport  Port=11  OutDataTypeStr=ValueType: mMconc
  His : Inport  Port=12  OutDataTypeStr=ValueType: mMconc
  Ile : Inport  Port=13  OutDataTypeStr=ValueType: mMconc
  Leu : Inport  Port=14  OutDataTypeStr=ValueType: mMconc
  Lys : Inport  Port=15  OutDataTypeStr=ValueType: mMconc
  Met : Inport  Port=16  OutDataTypeStr=ValueType: mMconc
  Phe : Inport  Port=17  OutDataTypeStr=ValueType: mMconc
  Pro : Inport  Port=18  OutDataTypeStr=ValueType: mMconc
  Ser : Inport  Port=19  OutDataTypeStr=ValueType: mMconc
  Thr : Inport  Port=20  OutDataTypeStr=ValueType: mMconc
  Trp : Inport  Port=21  OutDataTypeStr=ValueType: mMconc
  Tyr : Inport  Port=22  OutDataTypeStr=ValueType: mMconc
  Val : Inport  Port=23  OutDataTypeStr=ValueType: mMconc
  CMP : Inport  Port=24  OutDataTypeStr=ValueType: mMconc
  GMP : Inport  Port=25  OutDataTypeStr=ValueType: mMconc
  GMP1 : Inport  Port=26  OutDataTypeStr=ValueType: mMconc
  GMP2 : Inport  Port=27  OutDataTypeStr=ValueType: mMconc
  GMP3 : Inport  Port=28  OutDataTypeStr=ValueType: mMconc
  GMP4 : Inport  Port=29  OutDataTypeStr=ValueType: mMconc
  GMP5 : Inport  Port=30  OutDataTypeStr=ValueType: mMconc
  GMP6 : Inport  Port=31  OutDataTypeStr=ValueType: mMconc
  Bus Creator : BusCreator  Inputs=31  OutDataTypeStr=Bus: conc
      settings: InheritFromInputs=off
  conc : Outport  OutDataTypeStr=Bus: conc
  wires:
  Bus Creator/1 -> conc/1
  Xv/1 -> Bus Creator/1  "Xv"
  Glc/1 -> Bus Creator/2  "Glc"
  Lac/1 -> Bus Creator/3  "Lac"
  mAb/1 -> Bus Creator/4  "mAb"
  Ala/1 -> Bus Creator/5  "Glu"
  Arg/1 -> Bus Creator/6  "Gln"
  Asn/1 -> Bus Creator/7  "K"
  Asp/1 -> Bus Creator/8  "Na"
  Choline/1 -> Bus Creator/9  "NH4"
  Gly/1 -> Bus Creator/10  "Asp"
  Glu/1 -> Bus Creator/11  "Thr"
  His/1 -> Bus Creator/12  "Ser"
  Ile/1 -> Bus Creator/13  "Asn"
  Leu/1 -> Bus Creator/14  "GluAA"
  Lys/1 -> Bus Creator/15  "GlnAA"
  Met/1 -> Bus Creator/16  "Cys"
  Phe/1 -> Bus Creator/17  "Pro"
  Pro/1 -> Bus Creator/18  "Gly"
  Ser/1 -> Bus Creator/19  "Ala"
  Thr/1 -> Bus Creator/20  "Val"
  Trp/1 -> Bus Creator/21  "Met"
  Tyr/1 -> Bus Creator/22  "Cystine"
  Val/1 -> Bus Creator/23  "Ile"
  CMP/1 -> Bus Creator/24  "Leu"
  GMP/1 -> Bus Creator/25  "Tyr"
  GMP1/1 -> Bus Creator/26  "Phe"
  GMP2/1 -> Bus Creator/27  "Eth"
  GMP3/1 -> Bus Creator/28  "Trp"
  GMP4/1 -> Bus Creator/29  "Lys"
  GMP5/1 -> Bus Creator/30  "His"
  GMP6/1 -> Bus Creator/31  "Arg"

== system DT_Library/conc bus to conc array ==
  conc : Inport
  Concentration Split : $bdroot/Concentration Split  SystemSampleTime=-1  VariantActivationTime=update diagram  EmptyChoice=off  PassThrough=off  PassThroughVariantControl=(default)  EmptyChoiceVariantControl=(default)  AllowFlexibleInterface=on  Latency=0  AutoFrameSizeCalculation=off
  Mux : Mux  Inputs=31
  concArray : Outport
  wires:
  conc/1 -> Concentration Split/1
  Concentration Split/1 -> Mux/1
  Concentration Split/2 -> Mux/2
  Concentration Split/3 -> Mux/3
  Concentration Split/4 -> Mux/4
  Concentration Split/5 -> Mux/5
  Concentration Split/6 -> Mux/6
  Concentration Split/7 -> Mux/7
  Concentration Split/8 -> Mux/8
  Concentration Split/9 -> Mux/9
  Concentration Split/10 -> Mux/10
  Concentration Split/11 -> Mux/11
  Concentration Split/12 -> Mux/12
  Concentration Split/13 -> Mux/13
  Concentration Split/14 -> Mux/14
  Concentration Split/15 -> Mux/15
  Concentration Split/16 -> Mux/16
  Concentration Split/17 -> Mux/17
  Concentration Split/18 -> Mux/18
  Concentration Split/19 -> Mux/19
  Concentration Split/20 -> Mux/20
  Concentration Split/21 -> Mux/21
  Concentration Split/22 -> Mux/22
  Concentration Split/23 -> Mux/23
  Concentration Split/24 -> Mux/24
  Concentration Split/25 -> Mux/25
  Concentration Split/26 -> Mux/26
  Concentration Split/27 -> Mux/27
  Mux/1 -> concArray/1
  Concentration Split/28 -> Mux/28
  Concentration Split/29 -> Mux/29
  Concentration Split/30 -> Mux/30
  Concentration Split/31 -> Mux/31

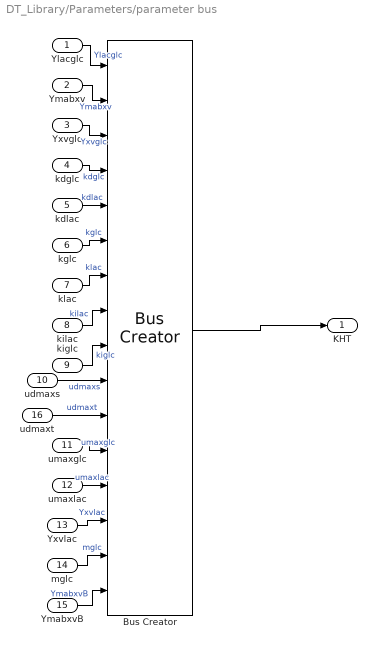
== system DT_Library/Parameters/parameter bus ==
  Ylacglc : Inport
  Ymabxv : Inport  Port=2
  Yxvglc : Inport  Port=3
  kdglc : Inport  Port=4
  kdlac : Inport  Port=5
  kglc : Inport  Port=6
  klac : Inport  Port=7
  kilac : Inport  Port=8
  kiglc : Inport  Port=9
  udmaxs : Inport  Port=10
  umaxglc : Inport  Port=11
  umaxlac : Inport  Port=12
  Yxvlac : Inport  Port=13
  mglc : Inport  Port=14
  YmabxvB : Inport  Port=15
  udmaxt : Inport  Port=16
  Bus Creator : BusCreator  Inputs=16  OutDataTypeStr=Bus: K
  KHT : Outport
  wires:
  Bus Creator/1 -> KHT/1
  Ylacglc/1 -> Bus Creator/1  "Ylacglc"
  Ymabxv/1 -> Bus Creator/2  "Ymabxv"
  Yxvglc/1 -> Bus Creator/3  "Yxvglc"
  kdglc/1 -> Bus Creator/4  "kdglc"
  kiglc/1 -> Bus Creator/9  "kiglc"
  kilac/1 -> Bus Creator/8  "kilac"
  kdlac/1 -> Bus Creator/5  "kdlac"
  klac/1 -> Bus Creator/7  "klac"
  kglc/1 -> Bus Creator/6  "kglc"
  udmaxs/1 -> Bus Creator/10  "udmaxs"
  umaxglc/1 -> Bus Creator/12  "umaxglc"
  umaxlac/1 -> Bus Creator/13  "umaxlac"
  Yxvlac/1 -> Bus Creator/14  "Yxvlac"
  mglc/1 -> Bus Creator/15  "mglc"
  YmabxvB/1 -> Bus Creator/16  "YmabxvB"
  udmaxt/1 -> Bus Creator/11  "udmaxt"

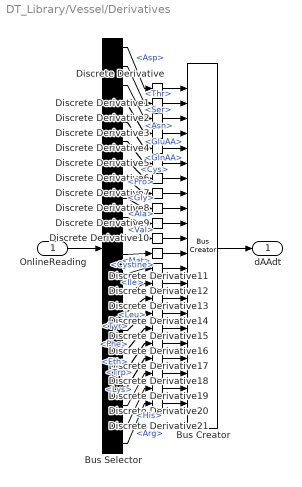
== system DT_Library/Vessel/Derivatives ==
  OnlineReading : Inport
  Bus Creator : BusCreator  Inputs=22  OutDataTypeStr=Bus: AA
      settings: InheritFromInputs=off
  Bus Selector : BusSelector  OutputSignals=Asp,Thr,Ser,Asn,GluAA,GlnAA,Cys,Pro,Gly,Ala,Val,Met,Cystine,Ile,Leu,Tyr,Phe,Eth,Trp,Lys,His,Arg
  Discrete Derivative{,1..21} (22 alike) : simulink/Discrete/Discrete Derivative  gainval=1.0  ICPrevScaledInput=0.0  OutMin=[]  OutMax=[]  OutDataType=fixdt(1, 16)  OutScaling=2^-10  DoSatur=off
  dAAdt : Outport  OutDataTypeStr=Bus: AA
  wires:
  OnlineReading/1 -> Bus Selector/1
  Bus Creator/1 -> dAAdt/1
  Bus Selector/1 -> Discrete Derivative/1  "<Asp>"
  Discrete Derivative/1 -> Bus Creator/1
  Discrete Derivative1/1 -> Bus Creator/2
  Bus Selector/2 -> Discrete Derivative1/1  "<Thr>"
  Discrete Derivative2/1 -> Bus Creator/3
  Bus Selector/3 -> Discrete Derivative2/1  "<Ser>"
  Discrete Derivative3/1 -> Bus Creator/4
  Bus Selector/4 -> Discrete Derivative3/1  "<Asn>"
  Discrete Derivative4/1 -> Bus Creator/5
  Bus Selector/5 -> Discrete Derivative4/1  "<GluAA>"
  Discrete Derivative5/1 -> Bus Creator/6
  Bus Selector/6 -> Discrete Derivative5/1  "<GlnAA>"
  Bus Selector/7 -> Discrete Derivative6/1  "<Cys>"
  Bus Selector/8 -> Discrete Derivative7/1  "<Pro>"
  Bus Selector/9 -> Discrete Derivative8/1  "<Gly>"
  Bus Selector/10 -> Discrete Derivative9/1  "<Ala>"
  Bus Selector/11 -> Discrete Derivative10/1  "<Val>"
  Bus Selector/12 -> Discrete Derivative11/1  "<Met>"
  Discrete Derivative21/1 -> Bus Creator/22
  Discrete Derivative20/1 -> Bus Creator/21
  Discrete Derivative19/1 -> Bus Creator/20
  Bus Selector/22 -> Discrete Derivative21/1  "<Arg>"
  Bus Selector/21 -> Discrete Derivative20/1  "<His>"
  Bus Selector/20 -> Discrete Derivative19/1  "<Lys>"
  Bus Selector/19 -> Discrete Derivative18/1  "<Trp>"
  Discrete Derivative18/1 -> Bus Creator/19
  Bus Selector/18 -> Discrete Derivative17/1  "<Eth>"
  Discrete Derivative17/1 -> Bus Creator/18
  Bus Selector/16 -> Discrete Derivative15/1  "<Tyr>"
  Bus Selector/17 -> Discrete Derivative16/1  "<Phe>"
  Bus Selector/15 -> Discrete Derivative14/1  "<Leu>"
  Bus Selector/14 -> Discrete Derivative13/1  "<Ile>"
  Bus Selector/13 -> Discrete Derivative12/1  "<Cystine>"
  Discrete Derivative16/1 -> Bus Creator/17
  Discrete Derivative15/1 -> Bus Creator/16
  Discrete Derivative14/1 -> Bus Creator/15
  Discrete Derivative13/1 -> Bus Creator/14
  Discrete Derivative12/1 -> Bus Creator/13
  Discrete Derivative11/1 -> Bus Creator/12
  Discrete Derivative10/1 -> Bus Creator/11
  Discrete Derivative9/1 -> Bus Creator/10
  Discrete Derivative8/1 -> Bus Creator/9
  Discrete Derivative7/1 -> Bus Creator/8
  Discrete Derivative6/1 -> Bus Creator/7

== system DT_Library/Vessel/GSM ==
  AAflux : Inport  OutDataTypeStr=Bus: AA
  OnlineReading : Inport  Port=2  OutDataTypeStr=Bus: conc
  GS model : MATLAB Function  TreatAsAtomicUnit=on
  gsrate : Outport  OutDataTypeStr=double
  wires:
  GS model/1(gsrate) -> gsrate/1
  AAflux/1 -> GS model/1(AAflux)
  OnlineReading/1 -> GS model/2(onlinereading)
  [phase] -> GS model/3(phase)
  [GSmode] -> GS model/4(GSmode)

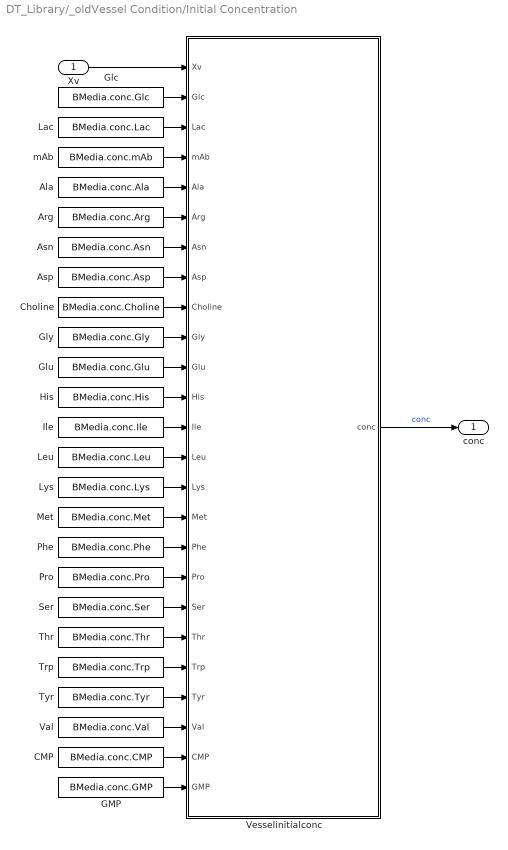
== system DT_Library/_oldVessel Condition/Initial Concentration ==
  Xv : Inport  OutDataTypeStr=ValueType: Xvconc
  Ala : Constant  Value=BMedia.conc.Ala  OutDataTypeStr=ValueType: mMconc
  Arg : Constant  Value=BMedia.conc.Arg  OutDataTypeStr=ValueType: mMconc
  Asn : Constant  Value=BMedia.conc.Asn  OutDataTypeStr=ValueType: mMconc
  Asp : Constant  Value=BMedia.conc.Asp  OutDataTypeStr=ValueType: mMconc
  CMP : Constant  Value=BMedia.conc.CMP  OutDataTypeStr=ValueType: mMconc
  Choline : Constant  Value=BMedia.conc.Choline  OutDataTypeStr=ValueType: mMconc
  GMP : Constant  Value=BMedia.conc.GMP  OutDataTypeStr=ValueType: mMconc
  Glc : Constant  Value=BMedia.conc.Glc  OutDataTypeStr=ValueType: gconc
  Glu : Constant  Value=BMedia.conc.Glu  OutDataTypeStr=ValueType: mMconc
  Gly : Constant  Value=BMedia.conc.Gly  OutDataTypeStr=ValueType: mMconc
  His : Constant  Value=BMedia.conc.His  OutDataTypeStr=ValueType: mMconc
  Ile : Constant  Value=BMedia.conc.Ile  OutDataTypeStr=ValueType: mMconc
  Lac : Constant  Value=BMedia.conc.Lac  OutDataTypeStr=ValueType: gconc
  Leu : Constant  Value=BMedia.conc.Leu  OutDataTypeStr=ValueType: mMconc
  Lys : Constant  Value=BMedia.conc.Lys  OutDataTypeStr=ValueType: mMconc
  Met : Constant  Value=BMedia.conc.Met  OutDataTypeStr=ValueType: mMconc
  Phe : Constant  Value=BMedia.conc.Phe  OutDataTypeStr=ValueType: mMconc
  Pro : Constant  Value=BMedia.conc.Pro  OutDataTypeStr=ValueType: mMconc
  Ser : Constant  Value=BMedia.conc.Ser  OutDataTypeStr=ValueType: mMconc
  Thr : Constant  Value=BMedia.conc.Thr  OutDataTypeStr=ValueType: mMconc
  Trp : Constant  Value=BMedia.conc.Trp  OutDataTypeStr=ValueType: mMconc
  Tyr : Constant  Value=BMedia.conc.Tyr  OutDataTypeStr=ValueType: mMconc
  Val : Constant  Value=BMedia.conc.Val  OutDataTypeStr=ValueType: mMconc
  Vesselinitialconc : Subsystem  TreatAsAtomicUnit=on
  mAb : Constant  Value=BMedia.conc.mAb  OutDataTypeStr=ValueType: gconc
  conc : Outport  OutDataTypeStr=Bus: conc
  wires:
  Xv/1 -> Vesselinitialconc/1(Xv)
  Glc/1 -> Vesselinitialconc/2(Glc)
  mAb/1 -> Vesselinitialconc/4(mAb)
  Lac/1 -> Vesselinitialconc/3(Lac)
  Asp/1 -> Vesselinitialconc/8(Asp)
  Ala/1 -> Vesselinitialconc/5(Ala)
  Arg/1 -> Vesselinitialconc/6(Arg)
  Asn/1 -> Vesselinitialconc/7(Asn)
  Choline/1 -> Vesselinitialconc/9(Choline)
  Gly/1 -> Vesselinitialconc/10(Gly)
  Glu/1 -> Vesselinitialconc/11(Glu)
  His/1 -> Vesselinitialconc/12(His)
  Ile/1 -> Vesselinitialconc/13(Ile)
  Leu/1 -> Vesselinitialconc/14(Leu)
  Lys/1 -> Vesselinitialconc/15(Lys)
  Met/1 -> Vesselinitialconc/16(Met)
  Phe/1 -> Vesselinitialconc/17(Phe)
  Pro/1 -> Vesselinitialconc/18(Pro)
  Ser/1 -> Vesselinitialconc/19(Ser)
  Thr/1 -> Vesselinitialconc/20(Thr)
  Trp/1 -> Vesselinitialconc/21(Trp)
  Tyr/1 -> Vesselinitialconc/22(Tyr)
  Val/1 -> Vesselinitialconc/23(Val)
  CMP/1 -> Vesselinitialconc/24(CMP)
  GMP/1 -> Vesselinitialconc/25(GMP)
  Vesselinitialconc/1(conc) -> conc/1  "conc"

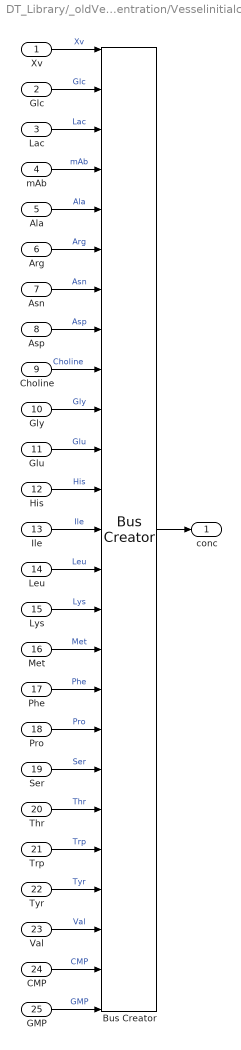
== system DT_Library/_oldVessel Condition/Initial Concentration/Vesselinitialconc ==
  Xv : Inport  OutDataTypeStr=ValueType: Xvconc
  Glc : Inport  Port=2  OutDataTypeStr=ValueType: gconc
  Lac : Inport  Port=3  OutDataTypeStr=ValueType: gconc
  mAb : Inport  Port=4  OutDataTypeStr=ValueType: gconc
  Ala : Inport  Port=5  OutDataTypeStr=ValueType: mMconc
  Arg : Inport  Port=6  OutDataTypeStr=ValueType: mMconc
  Asn : Inport  Port=7  OutDataTypeStr=ValueType: mMconc
  Asp : Inport  Port=8  OutDataTypeStr=ValueType: mMconc
  Choline : Inport  Port=9  OutDataTypeStr=ValueType: mMconc
  Gly : Inport  Port=10  OutDataTypeStr=ValueType: mMconc
  Glu : Inport  Port=11  OutDataTypeStr=ValueType: mMconc
  His : Inport  Port=12  OutDataTypeStr=ValueType: mMconc
  Ile : Inport  Port=13  OutDataTypeStr=ValueType: mMconc
  Leu : Inport  Port=14  OutDataTypeStr=ValueType: mMconc
  Lys : Inport  Port=15  OutDataTypeStr=ValueType: mMconc
  Met : Inport  Port=16  OutDataTypeStr=ValueType: mMconc
  Phe : Inport  Port=17  OutDataTypeStr=ValueType: mMconc
  Pro : Inport  Port=18  OutDataTypeStr=ValueType: mMconc
  Ser : Inport  Port=19  OutDataTypeStr=ValueType: mMconc
  Thr : Inport  Port=20  OutDataTypeStr=ValueType: mMconc
  Trp : Inport  Port=21  OutDataTypeStr=ValueType: mMconc
  Tyr : Inport  Port=22  OutDataTypeStr=ValueType: mMconc
  Val : Inport  Port=23  OutDataTypeStr=ValueType: mMconc
  CMP : Inport  Port=24  OutDataTypeStr=ValueType: mMconc
  GMP : Inport  Port=25  OutDataTypeStr=ValueType: mMconc
  Bus Creator : BusCreator  Inputs=Xv,Glc,Lac,mAb,Ala,Arg,Asn,Asp,Choline,Gly,Glu,His,Ile,Leu,Lys,Met,Phe,Pro,Ser,Thr,Trp,Tyr,Val,CMP,GMP  OutDataTypeStr=Bus: conc
  conc : Outport  OutDataTypeStr=Bus: conc
  wires:
  Bus Creator/1 -> conc/1
  Xv/1 -> Bus Creator/1  "Xv"
  Glc/1 -> Bus Creator/2  "Glc"
  Lac/1 -> Bus Creator/3  "Lac"
  mAb/1 -> Bus Creator/4  "mAb"
  Ala/1 -> Bus Creator/5  "Ala"
  Arg/1 -> Bus Creator/6  "Arg"
  Asn/1 -> Bus Creator/7  "Asn"
  Asp/1 -> Bus Creator/8  "Asp"
  Choline/1 -> Bus Creator/9  "Choline"
  Gly/1 -> Bus Creator/10  "Gly"
  Glu/1 -> Bus Creator/11  "Glu"
  His/1 -> Bus Creator/12  "His"
  Ile/1 -> Bus Creator/13  "Ile"
  Leu/1 -> Bus Creator/14  "Leu"
  Lys/1 -> Bus Creator/15  "Lys"
  Met/1 -> Bus Creator/16  "Met"
  Phe/1 -> Bus Creator/17  "Phe"
  Pro/1 -> Bus Creator/18  "Pro"
  Ser/1 -> Bus Creator/19  "Ser"
  Thr/1 -> Bus Creator/20  "Thr"
  Trp/1 -> Bus Creator/21  "Trp"
  Tyr/1 -> Bus Creator/22  "Tyr"
  Val/1 -> Bus Creator/23  "Val"
  CMP/1 -> Bus Creator/24  "CMP"
  GMP/1 -> Bus Creator/25  "GMP"
